simulink model "mazeBot"  (R2021b)
settings: Solver=FixedStepAuto  StartTime=0.0  StopTime=10.0  RelTol=1e-3  EnableMultiTasking=on
settings Model: ExtModeTrigDuration=2  Creator=romad  LastModifiedBy=romad
settings SolverCC: PositivePriorityOrder=on
settings OptimizationCC: EnhancedBackFolding=on  PassReuseOutputArgsAs=Individual arguments  ZeroExternalMemoryAtStartup=off  ZeroInternalMemoryAtStartup=off  MaxStackSize=64  OptimizeBlockOrder=speed  DifferentSizesBufferReuse=on  OptimizationCustomize=off  EfficientTunableParamExpr=on
settings DebuggingCC: ParameterTunabilityLossMsg=error
settings HardwareCC: ProdBitPerPointer=32  ProdBitPerSizeT=32  ProdBitPerPtrDiffT=32  ProdLargestAtomicInteger=Long  ProdWordSize=32  ProdHWDeviceType=ARM Compatible->ARM 9  UseEmbeddedCoderFeatures=off  UseSimulinkCoderFeatures=off
settings SFSimCC: MATLABDynamicMemAlloc=off
settings RTWCC: Description=Embedded Coder  SystemTargetFile=ert.tlc  HardwareBoard=LEGO MINDSTORMS EV3  TLCOptions="-aInlineSetEventsForThisBaseRateFcn=TLC_FALSE -aSuppressMultiTaskScheduler=TLC_FALSE  -aRateBasedStepFcn=0"  TemplateMakefile=ert_default_tmf  Toolchain=Sourcery G++ Lite v2009q3
settings CodeAppCC: ForceParamTrailComments=on  IgnoreCustomStorageClasses=off  OperatorAnnotations=on  SimulinkDataObjDesc=on  SFDataObjDesc=on  InsertBlockDesc=on
settings ERTTargetCC: SupportContinuousTime=on  SupportNonInlinedSFcns=on  SupportVariableSizeSignals=on  ExtModeTransport=2  ExtModeStaticAlloc=on  ExtModeMexFile=ext_xcp  ExtModeIntrfLevel=Level2 - Open

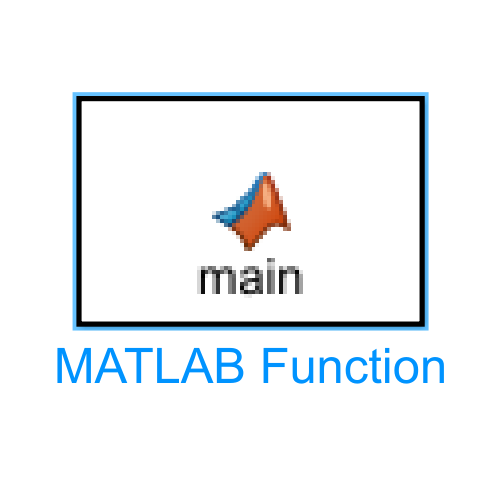
[thumbnail: Simulink's stored preview of the top-level diagram]
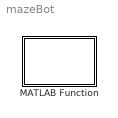
== system mazeBot ==
  MATLAB Function : MATLAB Function  TreatAsAtomicUnit=on

== matlab function mazeBot/MATLAB Function ==
function main()
    
    myrobot = legoev3('usb');   
    mA = motor(myrobot, 'A');
    mB = motor(myrobot, 'B');

    mA.Speed = 100;
    mB.Speed = 100;
    
    function moveForward()
        start(mA);
        start(mB);
    end
    function stopMotor()
        stop(mA, 1);
        stop(mB, 1); 
    end
    function turnRight()
        stop(mB, 1);
    end 
    function turnLeft()
        stop(mA, 1);
    end 
    
    sensor = sonicSensor(myrobot);
    distance = readDistance(sensor); %Ultrasonic sensor
    
    leftSensor = colorSensor(myrobot, 1);
    rightSensor = colorSensor(myrobot, 4);
    pause(0.5);
    while 1
        leftReflected = readLightIntensity(leftSensor, 'reflected');
        rightReflected = readLightIntensity(rightSensor, 'reflected');
        
        if leftReflected < 5
            turnLeft();
            pause(0.5);
        elseif rightReflected < 5
            turnRight();
            pause(0.5);
        else 
            moveForward();
        end

        pause(0.1);
    end

end
